simulink model "crazyflie"  (R2020a)
settings: Solver=FixedStepDiscrete  StartTime=0.0  StopTime=160  FixedStep=0.01  RelTol=1e-3
values from neighbouring files (symbols this model uses):
  alpha = 0.1    [Main_test.m]    (also in main_for_loading.m)
  Ts = 0.01    [Main_test.m]    (also in main_for_loading.m)
undefined symbols (not defined in the file or in its folder): DiscIntNeverNeededParam
settings Model: PauseTimes=7  Creator=Zrean  LastModifiedBy=hurr
settings DataIOCC: ReturnWorkspaceOutputs=off
settings OptimizationCC: DefaultParameterBehavior=Inlined  UseDivisionForNetSlopeComputation=on  UseFloatMulNetSlope=on  UseSpecifiedMinMax=on  InlineInvariantSignals=on  PassReuseOutputArgsAs=Individual arguments  ZeroExternalMemoryAtStartup=off  ZeroInternalMemoryAtStartup=off  NoFixptDivByZeroProtection=on  EfficientFloat2IntCast=on  LifeSpan=1  EfficientTunableParamExpr=on
settings DebuggingCC: AlgebraicLoopMsg=error  ParameterTunabilityLossMsg=error  ArithmeticOperatorsInVariantConditions=warning
settings HardwareCC: ProdBitPerPointer=32  ProdBitPerSizeT=32  ProdBitPerPtrDiffT=32  ProdLargestAtomicInteger=Long  ProdLargestAtomicFloat=Double  ProdWordSize=32  ProdHWDeviceType=ARM Compatible->ARM Cortex
settings SFSimCC: SimUseLocalCustomCode=off  MATLABDynamicMemAlloc=off  CustomCodeUndefinedFunction=UseInterfaceOnly
settings RTWCC: SystemTargetFile=ert.tlc  GenCodeOnly=on  TemplateMakefile=ert_default_tmf  GenerateReport=on  RTWUseLocalCustomCode=off  BuildConfiguration=Faster Runs  IncludeHyperlinkInReport=on  LaunchReport=on  GenerateTraceInfo=on  GenerateTraceReport=on  GenerateTraceReportSl=on  GenerateTraceReportSf=on  GenerateTraceReportEml=on  GenerateCodeMetricsReport=on
settings CodeAppCC: ForceParamTrailComments=on  IgnoreCustomStorageClasses=off  OperatorAnnotations=on  SimulinkDataObjDesc=on  SFDataObjDesc=on  MATLABFcnDesc=on  InsertBlockDesc=on  StateflowObjectComments=on  MATLABSourceComments=on
settings ERTTargetCC: TargetLangStandard=C99 (ISO)  MultiwordLength=2048  CombineSignalStateStructs=on  SuppressErrorStatus=on  SupportAbsoluteTime=off  SupportNonFinite=off  SupportComplex=off  InlinedParameterPlacement=NonHierarchical  ERTCustomFileTemplate=crazyflie_wrapper.tlc  ERTFilePackagingFormat=CompactWithDataFile
settings SimscapeCC: SimscapeNormalizeSystem=off

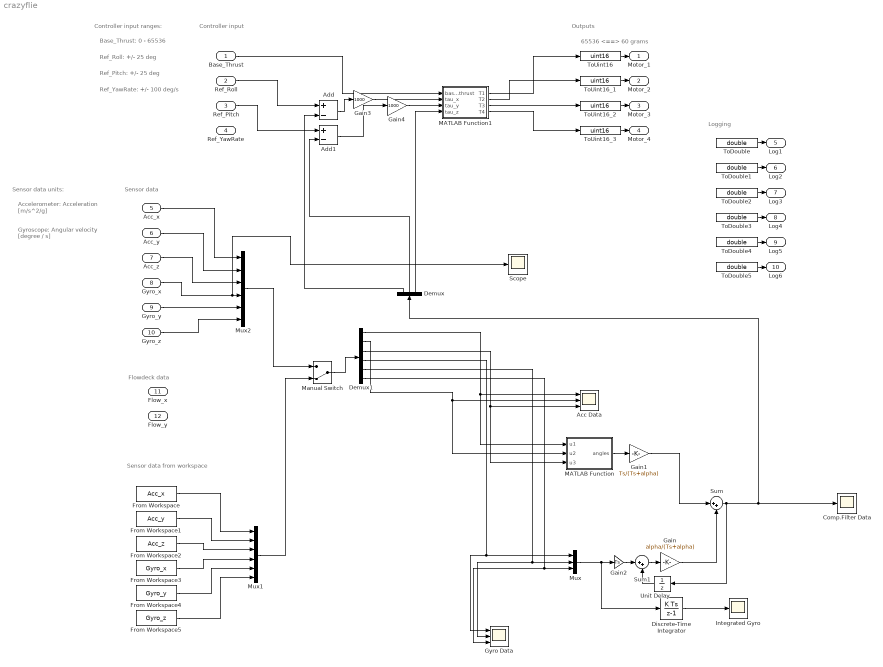
== system crazyflie ==
  note: 65536 <==> 60 grams
  note: Logging
  note: Outputs
  note: Sensor data
  note: Controller input
  note: Ref_Roll: +/- 25 deg
  note: Base_Thrust: 0 - 65536
  note: Ref_Pitch: +/- 25 deg
  note: Ref_YawRate: +/- 100 deg/s
  note: Controller input ranges:
  note: Gyroscope:
      | Angular velocity [degree / s]
  note: Accelerometer:
      | Acceleration [m/s^2/g]
  note: Sensor data units:
  note: Flowdeck data
  note: Sensor data from
      | workspace
  Base_Thrust : Inport  OutDataTypeStr=double
  Ref_Roll : Inport  Port=2  OutDataTypeStr=double
  Ref_Pitch : Inport  Port=3  OutDataTypeStr=double
  Ref_YawRate : Inport  Port=4  OutDataTypeStr=double
  Acc_x : Inport  Port=5  OutDataTypeStr=double  PortDimensions=1
  Acc_y : Inport  Port=6  OutDataTypeStr=double  PortDimensions=1
  Acc_z : Inport  Port=7  OutDataTypeStr=double  PortDimensions=1
  Gyro_x : Inport  Port=8  OutDataTypeStr=double  PortDimensions=1
  Gyro_y : Inport  Port=9  OutDataTypeStr=double  PortDimensions=1
  Gyro_z : Inport  Port=10  OutDataTypeStr=double  PortDimensions=1
  Flow_x : Inport  Port=11  OutDataTypeStr=int16  PortDimensions=1
  Flow_y : Inport  Port=12  OutDataTypeStr=int16  PortDimensions=1
  Acc Data : Scope  NumInputPorts=3
  Add : Sum  Inputs=+-
  Add1 : Sum  Inputs=+-
  Comp.Filter Data : Scope
  Demux : Demux  Outputs=3
  Demux1 : Demux  Outputs=6
  Discrete-Time Integrator : DiscreteIntegrator  SampleTime=Ts  ICPrevOutput=DiscIntNeverNeededParam  ICPrevScaledInput=DiscIntNeverNeededParam
  From Workspace : FromWorkspace  VariableName=Acc_x  OutDataTypeStr=double
  From Workspace1 : FromWorkspace  VariableName=Acc_y  OutDataTypeStr=double
  From Workspace2 : FromWorkspace  VariableName=Acc_z  OutDataTypeStr=double
  From Workspace3 : FromWorkspace  VariableName=Gyro_x  OutDataTypeStr=double
  From Workspace4 : FromWorkspace  VariableName=Gyro_y  OutDataTypeStr=double
  From Workspace5 : FromWorkspace  VariableName=Gyro_z  OutDataTypeStr=double
  Gain : Gain  Gain=alpha/(Ts+alpha)
  Gain1 : Gain  Gain=Ts/(Ts+alpha)
  Gain2 : Gain  Gain=Ts
  Gain3 : Gain  Gain=1000
  Gain4 : Gain  Gain=1000
  Gyro Data : Scope  NumInputPorts=3
  Integrated Gyro : Scope
  MATLAB Function : MATLAB Function  TreatAsAtomicUnit=on
  MATLAB Function1 : MATLAB Function  TreatAsAtomicUnit=on
  Manual Switch : ManualSwitch  CurrentSetting=0
  Mux : Mux  Inputs=3
  Mux1 : Mux  Inputs=6
  Mux2 : Mux  Inputs=6
  Scope : Scope
  Sum : Sum  Inputs=|++
  Sum1 : Sum  Inputs=|++
  ToDouble{,1..5} (6 alike) : DataTypeConversion  OutDataTypeStr=double  SaturateOnIntegerOverflow=on
  ToUint16 : DataTypeConversion  OutDataTypeStr=uint16  SaturateOnIntegerOverflow=on
  ToUint16_1 : DataTypeConversion  OutDataTypeStr=uint16  SaturateOnIntegerOverflow=on
  ToUint16_2 : DataTypeConversion  OutDataTypeStr=uint16  SaturateOnIntegerOverflow=on
  ToUint16_3 : DataTypeConversion  OutDataTypeStr=uint16  SaturateOnIntegerOverflow=on
  Unit Delay : UnitDelay  SampleTime=-1  HasFrameUpgradeWarning=on
  Motor_1 : Outport  OutDataTypeStr=uint16  VectorParamsAs1DForOutWhenUnconnected=off  LockScale=on
  Motor_2 : Outport  Port=2  OutDataTypeStr=uint16  VectorParamsAs1DForOutWhenUnconnected=off  LockScale=on
  Motor_3 : Outport  Port=3  OutDataTypeStr=uint16  VectorParamsAs1DForOutWhenUnconnected=off  LockScale=on
  Motor_4 : Outport  Port=4  OutDataTypeStr=uint16  VectorParamsAs1DForOutWhenUnconnected=off  LockScale=on
  Log1 : Outport  Port=5  OutDataTypeStr=double  VectorParamsAs1DForOutWhenUnconnected=off
  Log2 : Outport  Port=6  OutDataTypeStr=double  VectorParamsAs1DForOutWhenUnconnected=off
  Log3 : Outport  Port=7  OutDataTypeStr=double  VectorParamsAs1DForOutWhenUnconnected=off
  Log4 : Outport  Port=8  OutDataTypeStr=double  VectorParamsAs1DForOutWhenUnconnected=off
  Log5 : Outport  Port=9  OutDataTypeStr=double  VectorParamsAs1DForOutWhenUnconnected=off
  Log6 : Outport  Port=10  OutDataTypeStr=double  VectorParamsAs1DForOutWhenUnconnected=off
  wires:
  ToUint16/1 -> Motor_1/1
  ToUint16_1/1 -> Motor_2/1
  ToUint16_2/1 -> Motor_3/1
  ToUint16_3/1 -> Motor_4/1
  ToDouble/1 -> Log1/1
  ToDouble1/1 -> Log2/1
  ToDouble2/1 -> Log3/1
  ToDouble3/1 -> Log4/1
  ToDouble4/1 -> Log5/1
  ToDouble5/1 -> Log6/1
  From Workspace/1 -> Mux1/1
  From Workspace1/1 -> Mux1/2
  From Workspace2/1 -> Mux1/3
  From Workspace3/1 -> Mux1/4
  From Workspace4/1 -> Mux1/5
  From Workspace5/1 -> Mux1/6
  Mux/1 -> Gain2/1, Discrete-Time Integrator/1
  MATLAB Function/1(angles) -> Gain1/1
  Gain1/1 -> Sum/1
  Gain/1 -> Sum/2
  Sum/1 -> Demux/1, Comp.Filter Data/1, Unit Delay/1
  Discrete-Time Integrator/1 -> Integrated Gyro/1
  Sum1/1 -> Gain/1
  Unit Delay/1 -> Sum1/2
  Gain2/1 -> Sum1/1
  Base_Thrust/1 -> MATLAB Function1/1(base_thrust)
  Ref_Roll/1 -> Add/1
  Demux/1 -> Add/2
  Demux/2 -> Add1/2
  Ref_Pitch/1 -> Add1/1
  Add/1 -> Gain3/1
  Add1/1 -> Gain4/1
  Demux/3 -> MATLAB Function1/4(tau_z)
  MATLAB Function1/1(T1) -> ToUint16/1
  MATLAB Function1/2(T2) -> ToUint16_1/1
  MATLAB Function1/3(T3) -> ToUint16_2/1
  MATLAB Function1/4(T4) -> ToUint16_3/1
  Gain3/1 -> MATLAB Function1/2(tau_x)
  Gain4/1 -> MATLAB Function1/3(tau_y)
  Mux1/1 -> Manual Switch/2
  Acc_x/1 -> Mux2/1
  Acc_y/1 -> Mux2/2
  Acc_z/1 -> Mux2/3
  Gyro_x/1 -> Scope/1, Mux2/4
  Gyro_y/1 -> Mux2/5
  Gyro_z/1 -> Mux2/6
  Mux2/1 -> Manual Switch/1
  Manual Switch/1 -> Demux1/1
  Demux1/1 -> MATLAB Function/1(u1), Acc Data/1
  Demux1/2 -> MATLAB Function/2(u2), Acc Data/2
  Demux1/3 -> MATLAB Function/3(u3), Acc Data/3
  Demux1/4 -> Gyro Data/1, Mux/1
  Demux1/5 -> Gyro Data/2, Mux/2
  Demux1/6 -> Gyro Data/3, Mux/3

== matlab function crazyflie/MATLAB Function1 ==
  data: base_thrust input; T1 output; tau_x input; tau_y input; tau_z input; T2 output; T3 output; T4 output
function [T1,T2,T3,T4] = fcn(base_thrust,tau_x,tau_y,tau_z)

if tau_x > 0 
    xtemp3 = base_thrust;
    xtemp4 = base_thrust;
    xtemp12 = tau_x + xtemp3 + xtemp4;
    xtemp1 = xtemp12/2;
    xtemp2 = xtemp12/2;
else
    xtemp1 = base_thrust;
    xtemp2 = base_thrust;
    xtemp34 = -tau_x + xtemp1 + xtemp2;
    xtemp3 = xtemp34/2;
    xtemp4 = xtemp34/2;
end
if tau_y > 0
    ytemp2 = base_thrust;
    ytemp3 = base_thrust;
    ytemp14 = tau_y + ytemp2 + ytemp3;
    ytemp1 = ytemp14/2;
    ytemp4 = ytemp14/2;
else
    ytemp1 = base_thrust;
    ytemp4 = base_thrust;
    ytemp23 = -tau_y + ytemp1 + ytemp4;
    ytemp2 = ytemp23/2;
    ytemp3 = ytemp23/2;
end
T1 = xtemp1 + ytemp1;
T2 = xtemp2 + ytemp2;
T3 = xtemp3 + ytemp3;
T4 = xtemp4 + ytemp4;
end

== matlab function crazyflie/MATLAB Function ==
  data: u1 input; angles output; u2 input; u3 input
function angles = fcn(u1,u2,u3)
fx = u1/sqrt(u1^2 + u2^2 + u3^2);
fy = u2/sqrt(u1^2 + u2^2 + u3^2);
fz = u3/sqrt(u1^2 + u2^2 + u3^2);


angles = [atan2(fy,fz);atan2(-fx,sqrt(fy^2 + fz^2));0]*180/pi;
